simulink model "LinearIPS_Controller_Observer_Final"  (R2022a)
settings: Solver=FixedStepAuto  StartTime=0.0  StopTime=240  FixedStep=T  RelTol=1e-3
undefined symbols (not defined in the file): Ao, Bo, Co, DAS6036, Do, Measurement_Computing, PCI, QUAD04, T
libraries: sldrtlib x3
settings Model: SimulationMode=external  ExtModeTrigDuration=100000  Creator=Aaron Linares  LastModifiedBy=Mechatronics
settings SolverCC: AlgebraicLoopSolver=TrustRegion
settings DebuggingCC: UnconnectedInputMsg=warning  UnconnectedOutputMsg=warning  UnconnectedLineMsg=warning  SFMachineParentedDataDiag=warning
settings HardwareCC: ProdBitPerLong=64  ProdHWDeviceType=Intel->x86-64 (Linux 64)
settings RTWCC: Description=Simulink Desktop Real-Time  SystemTargetFile=sldrt.tlc  TemplateMakefile=sldrt.tmf  RTWCompilerOptimization=on  DLArmComputeVersion=19.05
settings CodeAppCC: MaxIdLength=95
settings SimulinkDesktopRealTimeCC: TargetLibSuffix=_sldrt.a  TargetPreCompLibLocation=C:\Program Files\MATLAB\R2022a\toolbox\sldrt\lib\win64

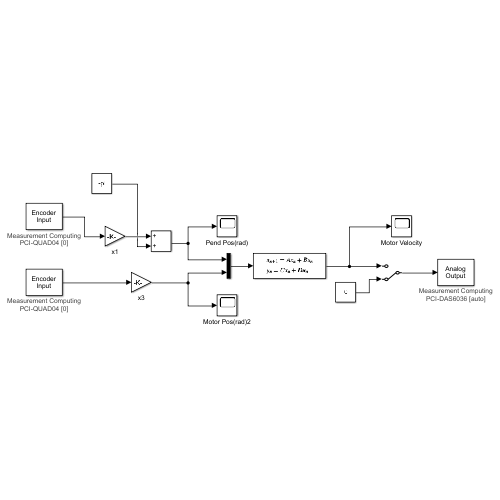
[thumbnail: Simulink's stored preview of the top-level diagram]
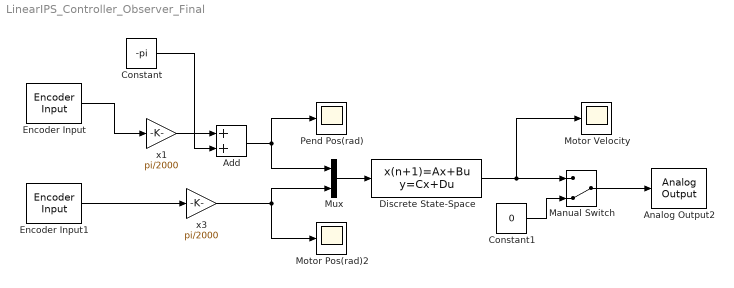
== system LinearIPS_Controller_Observer_Final ==
  Add : Sum
  Analog Output2 : sldrtlib/Analog Output  SampleTime=T  MaxMissedTicks=10  ShowMissedTicks=off  YieldWhenWaiting=off  DrvName=Measurement_Computing/PCI-DAS6036  DrvAddress=4294967295  DrvOptions=[255 0 0]  Channels=1  RangeMode=1  VoltRange=1  InitialValue=0  FinalValue=0
      settings: AttributesFormatString=Measurement Computing\nPCI-DAS6036 [auto]
  Constant : Constant  Value=-pi
  Constant1 : Constant  Value=0
  Discrete State-Space : DiscreteStateSpace  A=Ao  B=Bo  C=Co  D=Do  SampleTime=T
  Encoder Input : sldrtlib/Encoder Input  SampleTime=T  MaxMissedTicks=10  ShowMissedTicks=off  YieldWhenWaiting=off  DrvName=Measurement_Computing/PCI-QUAD04  DrvAddress=0  DrvOptions=zeros(1,0)  Channels=1  QuadMode=3  IndexPulse=3  InputFilter=Inf  DataType=1
      settings: AttributesFormatString=Measurement Computing\nPCI-QUAD04 [0]
  Encoder Input1 : sldrtlib/Encoder Input  SampleTime=T  MaxMissedTicks=10  ShowMissedTicks=off  YieldWhenWaiting=off  DrvName=Measurement_Computing/PCI-QUAD04  DrvAddress=0  DrvOptions=zeros(1,0)  Channels=2  QuadMode=3  IndexPulse=3  InputFilter=Inf  DataType=1
      settings: AttributesFormatString=Measurement Computing\nPCI-QUAD04 [0]
  Manual Switch : ManualSwitch  CurrentSetting=0
  Motor Pos(rad)2 : Scope
  Motor Velocity : Scope
  Mux : Mux  Inputs=2
  Pend Pos(rad) : Scope
  x1 : Gain  Gain=pi/2000
  x3 : Gain  Gain=pi/2000
  wires:
  x3/1 -> Mux/2, Motor Pos(rad)2/1
  Discrete State-Space/1 -> Motor Velocity/1, Manual Switch/1
  Add/1 -> Mux/1, Pend Pos(rad)/1
  Constant/1 -> Add/2
  x1/1 -> Add/1
  Constant1/1 -> Manual Switch/2
  Mux/1 -> Discrete State-Space/1
  Manual Switch/1 -> Analog Output2/1
  Encoder Input1/1 -> x3/1
  Encoder Input/1 -> x1/1
